simulink library "constXYZT_PlanarWave_cl"  (R2018b)
settings: Solver=VariableStepAuto  StartTime=0.0  StopTime=10.0  RelTol=1e-3
undefined symbols (not defined in the file): env
libraries: planarWaveModel_ul x1
settings Model: Creator=mcobb  LastModifiedBy=jcreed2

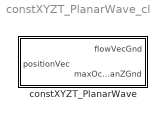
== system constXYZT_PlanarWave_cl ==
  constXYZT_PlanarWave : Subsystem

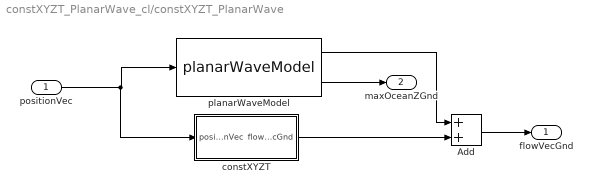
== system constXYZT_PlanarWave_cl/constXYZT_PlanarWave ==
  positionVec : Inport
  Add : Sum
  constXYZT : Subsystem  mask{constXYZT=env.water}
      mask prompts: constXYZT "env.constXYZT Object"
  planarWaveModel : planarWaveModel_ul/planarWaveModel  SystemSampleTime=-1
  flowVecGnd : Outport
  maxOceanZGnd : Outport  Port=2
  wires:
  positionVec/1 -> constXYZT/1(positionVec), planarWaveModel/1
  planarWaveModel/2 -> maxOceanZGnd/1
  Add/1 -> flowVecGnd/1
  constXYZT/1(flowVecGnd) -> Add/2
  planarWaveModel/1 -> Add/1

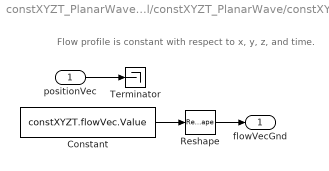
== system constXYZT_PlanarWave_cl/constXYZT_PlanarWave/constXYZT ==
  note: Flow profile is constant with respect to x, y, z, and time.
  positionVec : Inport
  Constant : Constant  Value=constXYZT.flowVec.Value
  Reshape : Reshape  OutputDimensionality=Column vector (2-D)
  Terminator : Terminator
  flowVecGnd : Outport
  wires:
  positionVec/1 -> Terminator/1
  Constant/1 -> Reshape/1
  Reshape/1 -> flowVecGnd/1
